simulink model "model"  (R2017b)
settings: Solver=VariableStepAuto  StartTime=0.0  StopTime=10.0  RelTol=1e-3
undefined symbols (not defined in the file or in its folder): bf, br, ca, J, lf, lr, mv, rho
settings Model: Creator=chitr  LastModifiedBy=chitr

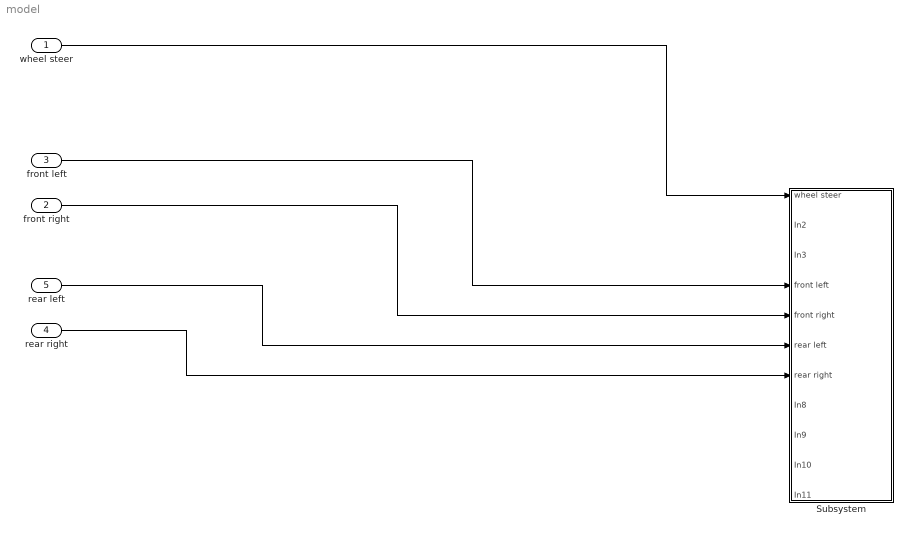
== system model ==
  wheel steer : Inport
  front right : Inport  Port=2
  front left : Inport  Port=3
  rear right : Inport  Port=4
  rear left : Inport  Port=5
  Subsystem : Subsystem
  wires:
  wheel steer/1 -> Subsystem/1(wheel steer)
  front left/1 -> Subsystem/4(front left)
  front right/1 -> Subsystem/5(front right)
  rear left/1 -> Subsystem/6(rear left)
  rear right/1 -> Subsystem/7(rear right)

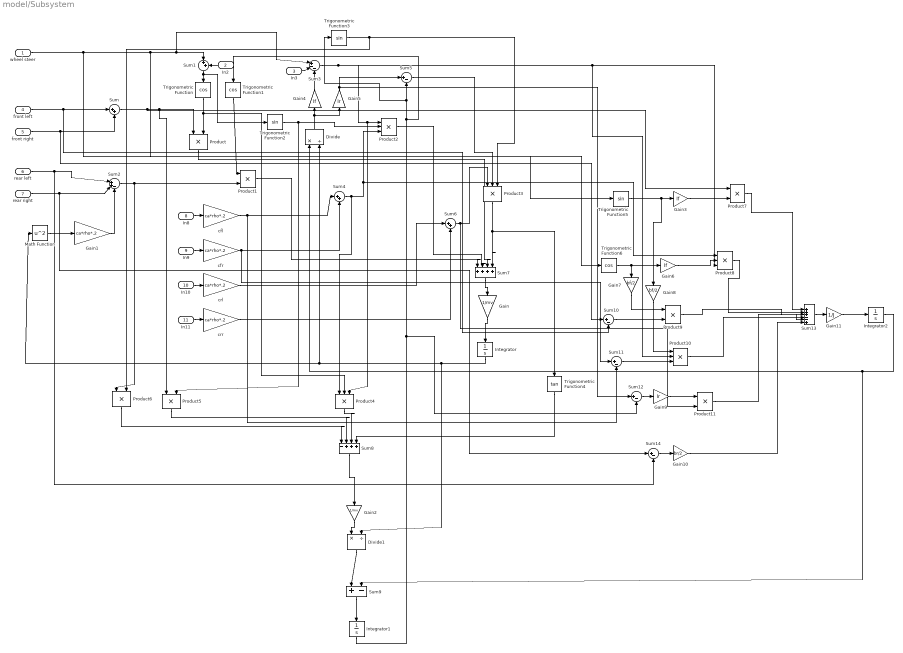
== system model/Subsystem ==
  wheel steer : Inport
  In2 : Inport  Port=2
  In3 : Inport  Port=3
  front left : Inport  Port=4
  front right : Inport  Port=5
  rear left : Inport  Port=6
  rear right : Inport  Port=7
  In8 : Inport  Port=8
  In9 : Inport  Port=9
  In10 : Inport  Port=10
  In11 : Inport  Port=11
  Divide : Product  Inputs=*/
  Divide1 : Product  Inputs=*/
  Gain : Gain  Gain=1/mv
  Gain1 : Gain  Gain=ca*rho*.2
  Gain10 : Gain  Gain=br/2
  Gain11 : Gain  Gain=1/J
  Gain2 : Gain  Gain=1/mv
  Gain3 : Gain  Gain=lf
  Gain4 : Gain  Gain=lf
  Gain5 : Gain  Gain=lr
  Gain6 : Gain  Gain=lf
  Gain7 : Gain  Gain=bf/2
  Gain8 : Gain  Gain=bf/2
  Gain9 : Gain  Gain=lr
  Integrator : Integrator
  Integrator1 : Integrator
  Integrator2 : Integrator
  Math Function : Math  Operator=square  SaturateOnIntegerOverflow=on
  Product{,1,5..7,9,11} (7 alike) : Product
  Product{2..4,8,10} (5 alike) : Product  Inputs=3
  Sum{,1,4,6} (4 alike) : Sum  Inputs=|++
  Sum{5,9..12,14} (6 alike) : Sum  Inputs=|+-
  Sum13 : Sum  Inputs=|+++--+
  Sum2 : Sum  Inputs=|++-
  Sum3 : Sum  Inputs=|+--
  Sum7 : Sum  Inputs=|++++
  Sum8 : Sum  Inputs=|-+++
  Trigonometric Function : Trigonometry  Operator=cos
  Trigonometric Function1 : Trigonometry  Operator=cos
  Trigonometric Function2 : Trigonometry
  Trigonometric Function3 : Trigonometry
  Trigonometric Function4 : Trigonometry  Operator=tan
  Trigonometric Function5 : Trigonometry
  Trigonometric Function6 : Trigonometry  Operator=cos
  cfl : Gain  Gain=ca*rho*.2
  cfr : Gain  Gain=ca*rho*.2
  crl : Gain  Gain=ca*rho*.2
  crr : Gain  Gain=ca*rho*.2
  wires:
  Divide/1 -> Gain5/1, Gain4/1
  Sum10/1 -> Product9/2
  Trigonometric Function2/1 -> Product5/2, Product2/2
  Gain5/1 -> Sum12/1, Sum5/1
  Gain11/1 -> Integrator2/1
  Sum2/1 -> Product6/1, Product1/2
  crr/1 -> Sum6/2
  cfl/1 -> Sum11/2, Sum4/1
  front right/1 -> Sum10/1, Sum/2
  Product5/1 -> Sum8/2
  Product1/1 -> Sum7/1
  Math Function/1 -> Gain1/1
  Gain/1 -> Integrator/1
  Sum7/1 -> Gain/1
  crl/1 -> Sum6/1
  Sum6/1 -> Product11/2, Product3/1
  rear left/1 -> Sum14/2, Sum2/1
  cfr/1 -> Sum11/1, Sum4/2
  Trigonometric Function/1 -> Product4/2, Product/2
  Sum8/1 -> Gain2/1
  front left/1 -> Sum10/2, Sum/1
  Product6/1 -> Sum8/1
  wheel steer/1 -> Trigonometric Function6/1, Trigonometric Function5/1, Sum3/1, Sum1/1
  Product3/1 -> Trigonometric Function4/1, Sum7/4
  Gain4/1 -> Sum3/3
  Integrator/1 -> Divide1/2, Divide/2, Math Function/1
  Sum5/1 -> Product3/2
  Sum1/1 -> Trigonometric Function2/1, Trigonometric Function/1
  Product2/1 -> Sum7/2
  Gain1/1 -> Sum2/3
  Integrator1/1 -> Sum12/2, Trigonometric Function1/1, Trigonometric Function3/1, Sum5/2
  Trigonometric Function1/1 -> Product1/1
  Product/1 -> Sum7/3
  Trigonometric Function4/1 -> Sum8/4
  rear right/1 -> Sum14/1, Sum2/2
  Product7/1 -> Sum13/1
  Sum13/1 -> Gain11/1
  Product4/1 -> Sum8/3
  Sum14/1 -> Gain10/1
  Gain8/1 -> Product10/1
  Sum11/1 -> Product10/3
  Sum9/1 -> Integrator1/1
  Gain9/1 -> Product11/1
  Product11/1 -> Sum13/5
  Gain3/1 -> Product7/2
  Product10/1 -> Sum13/4
  Gain2/1 -> Divide1/1
  Sum3/1 -> Product10/2, Product8/3, Product4/3, Product2/1
  Integrator2/1 -> Sum9/2, Divide/1
  Divide1/1 -> Sum9/1
  Gain7/1 -> Product9/1
  Product9/1 -> Sum13/3
  Gain6/1 -> Product8/2
  Sum4/1 -> Product4/1, Product8/1, Product2/3
  Product8/1 -> Sum13/2
  Trigonometric Function6/1 -> Gain6/1, Gain7/1
  Sum12/1 -> Gain9/1
  Trigonometric Function5/1 -> Gain8/1, Gain3/1
  In9/1 -> cfr/1
  In8/1 -> cfl/1
  In3/1 -> Sum3/2
  In2/1 -> Sum1/2
  In10/1 -> crl/1
  In11/1 -> crr/1
  Gain10/1 -> Sum13/6
  Sum/1 -> Product7/1, Product5/1, Product/1
  Trigonometric Function3/1 -> Product6/2, Product3/3
